simulink model "controllore_coppia"  (R2020a)
settings: Solver=VariableStepAuto  StartTime=0.0  StopTime=10.0  RelTol=1e-3
values from neighbouring files (symbols this model uses):
  g = 9.81    [dati_tesi_modellosimulink.m]
  L = 0.3    [dati_tesi_modellosimulink.m]
  Lc = L/2    (= 0.15)    [dati_tesi_modellosimulink.m]
  M = 4    [dati_tesi_modellosimulink.m]
  mc = 0    [dati_tesi_modellosimulink.m]
libraries: fuzblock x7, simulink x2, simulink_extras x2, cstblocks x1
settings Model: Creator=laura  LastModifiedBy=laura

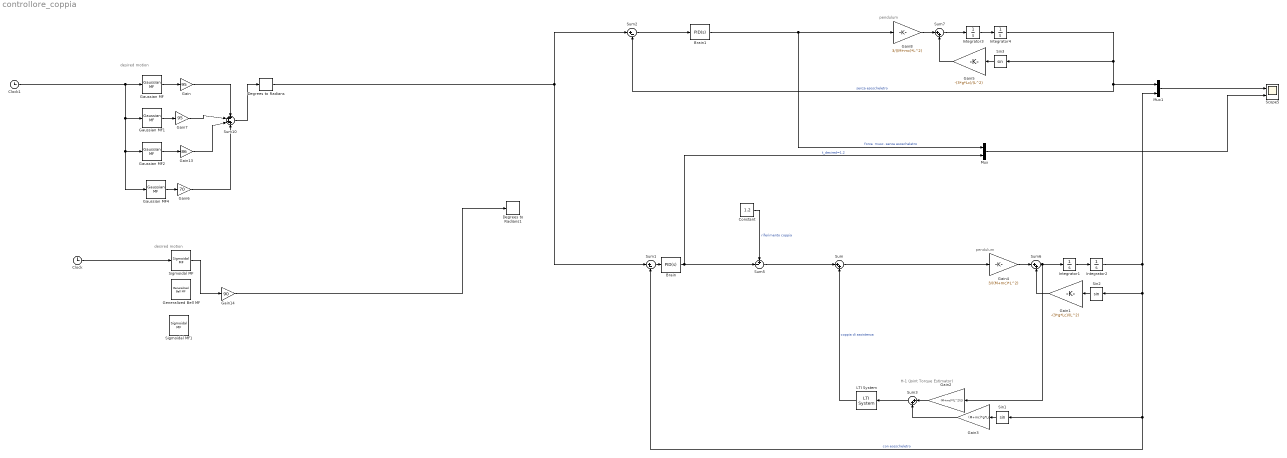
== system controllore_coppia ==
  note: desired motion
  note: H-1 (Joint Torque Estimator)
  note: pendulum
  note: desired motion
  note: pendulum
  Brain : simulink/Continuous/PID Controller  Controller=PID  Form=Parallel  TimeDomain=Continuous-time  UseExternalTs=off  SampleTime=-1  IntegratorMethod=Forward Euler  FilterMethod=Forward Euler  ControllerParametersSource=internal  P=20.396  I=105.7651  D=6.3413  UseFilter=on  N=150.7964  TunerSelectOption=Transfer Function Based (PID Tuner App)  InitialConditionSource=internal  InitialConditionForIntegrator=0  InitialConditionForFilter=0  DifferentiatorICPrevScaledInput=0  ExternalReset=none  TrackingMode=off  Kt=1  LimitOutput=off  UpperSaturationLimit=inf  LowerSaturationLimit=-inf  LinearizeAsGain=on  AntiWindupMode=none  Kb=1  POutMin=[]  POutMax=[]  IOutMin=[]  IOutMax=[]  DOutMin=[]  DOutMax=[]  NOutMin=[]  NOutMax=[]  SumOutMin=[]  SumOutMax=[]  SaturationOutMin=[]  SaturationOutMax=[]  PParamMin=[]  PParamMax=[]  IParamMin=[]  IParamMax=[]  DParamMin=[]  DParamMax=[]  NParamMin=[]  NParamMax=[]  KbParamMin=[]  KbParamMax=[]  KtParamMin=[]  KtParamMax=[]  KbOutMin=[]  KbOutMax=[]  KtOutMin=[]  KtOutMax=[]  IntegratorOutMin=[]  IntegratorOutMax=[]  FilterOutMin=[]  FilterOutMax=[]  SumI1OutMin=[]  SumI1OutMax=[]  SumI2OutMin=[]  SumI2OutMax=[]  SumI3OutMin=[]  SumI3OutMax=[]  SumI4OutMin=[]  SumI4OutMax=[]  SumDOutMin=[]  SumDOutMax=[]  DifferentiatorOutMin=[]  DifferentiatorOutMax=[]  FilterDiffOutCoefMin=[]  FilterDiffOutCoefMax=[]  ReciprocalOutMin=[]  ReciprocalOutMax=[]  SumDenOutMin=[]  SumDenOutMax=[]  SumNumOutMin=[]  SumNumOutMax=[]  DivideOutMin=[]  DivideOutMax=[]  UdiffTsProdOutMin=[]  UdiffTsProdOutMax=[]  NTsProdOutMin=[]  NTsProdOutMax=[]  UintegralTsProdOutMin=[]  UintegralTsProdOutMax=[]  UngainTsProdOutMin=[]  UngainTsProdOutMax=[]  IntegratorContinuousStateAttributes=''  IntegratorStateMustResolveToSignalObject=off  IntegratorRTWStateStorageClass=Auto  FilterContinuousStateAttributes=''  FilterStateMustResolveToSignalObject=off  FilterRTWStateStorageClass=Auto  ParallelPVariant=InternalParameters  IdealPVariant=Disabled  IVariant=InternalParameters  DVariant=InternalParameters  IntegratorVariant=Continuous  SatVariant=Disabled  AWVariant=Passthrough  PCopyVariant=Disabled  TRVariant=Disabled  FdbkBlocksVariant=Forward  IdealPFdbkVariant=Disabled  SatFdbkVariant=Disabled  DerivativeFilterVariant=ContFilter  NVariant=InternalParameters  NCopyVariant=Disabled  FilterICVariant=InternalICsFilter  IntegratorICVariant=InternalICs  ExternalResetVariant=Disabled  TRSumVariant=Passthrough  SumFdbkVariant=Disabled  SumVariant=Sum_PID  TsampFilterVariant=InternalTs  TsampNgainVariant=Passthrough  TsampIntegralVariant=Passthrough
  Brain1 : simulink/Continuous/PID Controller  Controller=PID  Form=Parallel  TimeDomain=Continuous-time  UseExternalTs=off  SampleTime=-1  IntegratorMethod=Forward Euler  FilterMethod=Forward Euler  ControllerParametersSource=internal  P=20.396  I=105.7651  D=6.3413  UseFilter=on  N=150.7964  TunerSelectOption=Transfer Function Based (PID Tuner App)  InitialConditionSource=internal  InitialConditionForIntegrator=0  InitialConditionForFilter=0  DifferentiatorICPrevScaledInput=0  ExternalReset=none  TrackingMode=off  Kt=1  LimitOutput=off  UpperSaturationLimit=inf  LowerSaturationLimit=-inf  LinearizeAsGain=on  AntiWindupMode=none  Kb=1  POutMin=[]  POutMax=[]  IOutMin=[]  IOutMax=[]  DOutMin=[]  DOutMax=[]  NOutMin=[]  NOutMax=[]  SumOutMin=[]  SumOutMax=[]  SaturationOutMin=[]  SaturationOutMax=[]  PParamMin=[]  PParamMax=[]  IParamMin=[]  IParamMax=[]  DParamMin=[]  DParamMax=[]  NParamMin=[]  NParamMax=[]  KbParamMin=[]  KbParamMax=[]  KtParamMin=[]  KtParamMax=[]  KbOutMin=[]  KbOutMax=[]  KtOutMin=[]  KtOutMax=[]  IntegratorOutMin=[]  IntegratorOutMax=[]  FilterOutMin=[]  FilterOutMax=[]  SumI1OutMin=[]  SumI1OutMax=[]  SumI2OutMin=[]  SumI2OutMax=[]  SumI3OutMin=[]  SumI3OutMax=[]  SumI4OutMin=[]  SumI4OutMax=[]  SumDOutMin=[]  SumDOutMax=[]  DifferentiatorOutMin=[]  DifferentiatorOutMax=[]  FilterDiffOutCoefMin=[]  FilterDiffOutCoefMax=[]  ReciprocalOutMin=[]  ReciprocalOutMax=[]  SumDenOutMin=[]  SumDenOutMax=[]  SumNumOutMin=[]  SumNumOutMax=[]  DivideOutMin=[]  DivideOutMax=[]  UdiffTsProdOutMin=[]  UdiffTsProdOutMax=[]  NTsProdOutMin=[]  NTsProdOutMax=[]  UintegralTsProdOutMin=[]  UintegralTsProdOutMax=[]  UngainTsProdOutMin=[]  UngainTsProdOutMax=[]  IntegratorContinuousStateAttributes=''  IntegratorStateMustResolveToSignalObject=off  IntegratorRTWStateStorageClass=Auto  FilterContinuousStateAttributes=''  FilterStateMustResolveToSignalObject=off  FilterRTWStateStorageClass=Auto  ParallelPVariant=InternalParameters  IdealPVariant=Disabled  IVariant=InternalParameters  DVariant=InternalParameters  IntegratorVariant=Continuous  SatVariant=Disabled  AWVariant=Passthrough  PCopyVariant=Disabled  TRVariant=Disabled  FdbkBlocksVariant=Forward  IdealPFdbkVariant=Disabled  SatFdbkVariant=Disabled  DerivativeFilterVariant=ContFilter  NVariant=InternalParameters  NCopyVariant=Disabled  FilterICVariant=InternalICsFilter  IntegratorICVariant=InternalICs  ExternalResetVariant=Disabled  TRSumVariant=Passthrough  SumFdbkVariant=Disabled  SumVariant=Sum_PID  TsampFilterVariant=InternalTs  TsampNgainVariant=Passthrough  TsampIntegralVariant=Passthrough
  Clock : Clock
  Clock1 : Clock
  Constant : Constant  Value=1.2
  Degrees to Radians : simulink_extras/Transformations/Degrees to Radians
  Degrees to Radians1 : simulink_extras/Transformations/Degrees to Radians
  Gain : Gain  Gain=95
  Gain1 : Gain  Gain=-(3*g*Lc)/(L^2)
  Gain13 : Gain  Gain=86
  Gain14 : Gain  Gain=90
  Gain2 : Gain  Gain=(M+mc)*(L^2)/3
  Gain3 : Gain  Gain=(M+mc)*g*Lc
  Gain4 : Gain  Gain=3/((M+mc)*L^2)
  Gain5 : Gain  Gain=-(3*g*Lc)/(L^2)
  Gain6 : Gain  Gain=70
  Gain7 : Gain  Gain=95
  Gain8 : Gain  Gain=3/((M+mc)*L^2)
  Gaussian MF : fuzblock/Membership  Functions/Gaussian MF  sigma=0.4  mu=1.78
      settings: SourceProductBaseCode=FL
  Gaussian MF1 : fuzblock/Membership  Functions/Gaussian MF  sigma=0.4  mu=7
      settings: SourceProductBaseCode=FL
  Gaussian MF2 : fuzblock/Membership  Functions/Gaussian MF  sigma=0.38  mu=3.42
      settings: SourceProductBaseCode=FL
  Gaussian MF4 : fuzblock/Membership  Functions/Gaussian MF  sigma=0.32  mu=2.63
      settings: SourceProductBaseCode=FL
  Generalized Bell MF : fuzblock/Membership  Functions/Generalized Bell MF  a=1.5  b=4  c=6
      settings: SourceProductBaseCode=FL
  Integrator{1..4} (4 alike) : Integrator
  LTI System : cstblocks/LTI System  sys=C  IC=[]
  Mux : Mux  Inputs=2
  Mux1 : Mux  Inputs=2
  Scope5 : Scope  NumInputPorts=2
  Sigmoidal MF : fuzblock/Membership  Functions/Sigmoidal MF  a=4  c=5
      settings: SourceProductBaseCode=FL
  Sigmoidal MF1 : fuzblock/Membership  Functions/Sigmoidal MF  a=-4  c=5
      settings: SourceProductBaseCode=FL
  Sin1 : Trigonometry
  Sin2 : Trigonometry
  Sin3 : Trigonometry
  Sum{,3,6..7} (4 alike) : Sum  Inputs=|++
  Sum1 : Sum  Inputs=|+-
  Sum10 : Sum  Inputs=++++
  Sum2 : Sum  Inputs=|+-
  Sum5 : Sum  Inputs=+-|
  wires:
  Brain/1 -> Sum5/2, Mux/2  "t_desired=1.2"
  Sum5/1 -> Sum/1
  Clock/1 -> Sigmoidal MF/1
  Gain1/1 -> Sum6/2
  Constant/1 -> Sum5/1  "riferimento coppia"
  Sigmoidal MF/1 -> Gain14/1
  Sum7/1 -> Integrator3/1
  Sin3/1 -> Gain5/1
  Sum/1 -> Gain4/1
  Sin1/1 -> Gain3/1
  Integrator2/1 -> Mux1/2, Sum1/2, Sin1/1, Sin2/1  "con eosscheletro"
  Integrator1/1 -> Integrator2/1
  Gain2/1 -> Sum3/1
  Brain1/1 -> Mux/1, Gain8/1  "forza  musc. senza esoscheletro"
  Integrator4/1 -> Sum2/2, Mux1/1, Sin3/1  "senza esoscheletro"
  Sum1/1 -> Brain/1
  Gain5/1 -> Sum7/2
  Clock1/1 -> Gaussian MF4/1, Gaussian MF2/1, Gaussian MF1/1, Gaussian MF/1
  Integrator3/1 -> Integrator4/1
  Gaussian MF4/1 -> Gain6/1
  Gain/1 -> Sum10/1
  Sum6/1 -> Gain2/1, Integrator1/1
  LTI System/1 -> Sum/2  "coppia di assistenza"
  Sum3/1 -> LTI System/1
  Gain4/1 -> Sum6/1
  Gain13/1 -> Sum10/3
  Gain14/1 -> Degrees to Radians1/1
  Gain3/1 -> Sum3/2
  Degrees to Radians/1 -> Sum1/1, Sum2/1
  Gaussian MF2/1 -> Gain13/1
  Gaussian MF/1 -> Gain/1
  Sin2/1 -> Gain1/1
  Gain6/1 -> Sum10/4
  Gain8/1 -> Sum7/1
  Gain7/1 -> Sum10/2
  Gaussian MF1/1 -> Gain7/1
  Sum2/1 -> Brain1/1
  Sum10/1 -> Degrees to Radians/1
  Mux/1 -> Scope5/2
  Mux1/1 -> Scope5/1
